simulink library "starslibMathOperations"  (R2024b)
settings: Solver=ode45  StartTime=0.0  StopTime=10.0  RelTol=1e-3  EnableMultiTasking=on
libraries: $bdroot x8
(part 2 of 2)

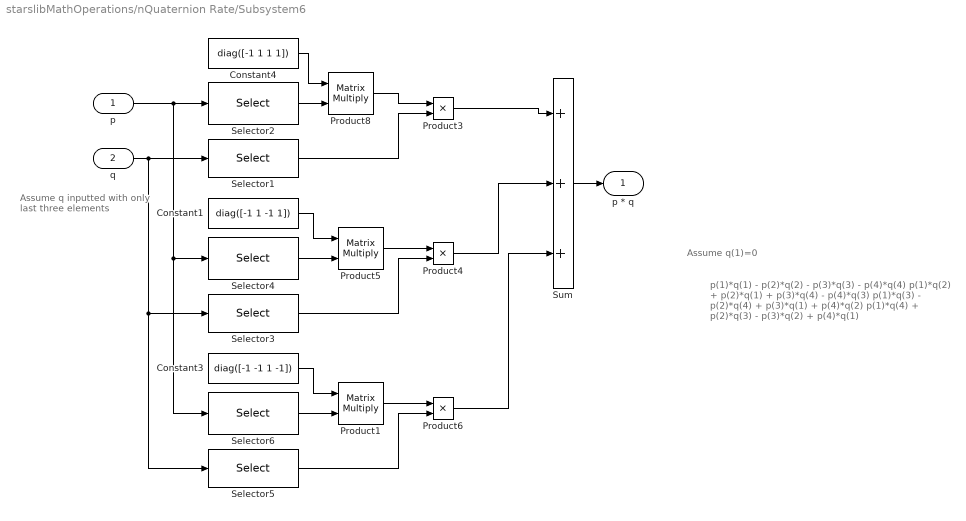
== system starslibMathOperations/nQuaternion Rate/Subsystem6 ==
  note: Assume q
      | inputted with only
      | last three elements
  note: Assume q(1)=0
  note: p(1)*q(1) - p(2)*q(2) - p(3)*q(3) - p(4)*q(4)
      |
      | p(1)*q(2) + p(2)*q(1) + p(3)*q(4) - p(4)*q(3)
      |
      | p(1)*q(3) - p(2)*q(4) + p(3)*q(1) + p(4)*q(2)
      |
      | p(1)*q(4) + p(2)*q(3) - p(3)*q(2) + p(4)*q(1)
  p : Inport  PortDimensions=[4,nQuat]
  q : Inport  Port=2  PortDimensions=[3,nQuat]
  Constant1 : Constant  Value=diag([-1 1 -1 1])  VectorParams1D=off
  Constant3 : Constant  Value=diag([-1 -1 1 -1])  VectorParams1D=off
  Constant4 : Constant  Value=diag([-1 1 1 1])  VectorParams1D=off
  Product1 : Product  Multiplication=Matrix(*)  RndMeth=Zero
  Product3 : Product  RndMeth=Zero
  Product4 : Product  RndMeth=Zero
  Product5 : Product  Multiplication=Matrix(*)  RndMeth=Zero
  Product6 : Product  RndMeth=Zero
  Product8 : Product  Multiplication=Matrix(*)  RndMeth=Zero
  Selector1 : Selector  NumberOfDimensions=2  InputPortWidth=3  IndexOptions=Index vector (dialog),Select all  Indices=[1 1 2 3],1  OutputSizes=1,1
  Selector2 : Selector  NumberOfDimensions=2  InputPortWidth=3  IndexOptions=Index vector (dialog),Select all  Indices=[2 1 1 1],1  OutputSizes=1,1
  Selector3 : Selector  NumberOfDimensions=2  InputPortWidth=3  IndexOptions=Index vector (dialog),Select all  Indices=[2 3 3 2],1  OutputSizes=1,1
  Selector4 : Selector  NumberOfDimensions=2  InputPortWidth=3  IndexOptions=Index vector (dialog),Select all  Indices=[3 3 2 2],1  OutputSizes=1,1
  Selector5 : Selector  NumberOfDimensions=2  InputPortWidth=3  IndexOptions=Index vector (dialog),Select all  Indices=[3 2 1 1],1  OutputSizes=1,1
  Selector6 : Selector  NumberOfDimensions=2  InputPortWidth=3  IndexOptions=Index vector (dialog),Select all  Indices=[4 4 4 3],1  OutputSizes=1,1
  Sum : Sum  Inputs=+++
  p * q : Outport  PortDimensions=[4,nQuat]
  wires:
  Constant4/1 -> Product8/1
  Product8/1 -> Product3/1
  Selector2/1 -> Product8/2
  Sum/1 -> p * q/1
  q/1 -> Selector5/1, Selector3/1, Selector1/1
  p/1 -> Selector6/1, Selector4/1, Selector2/1
  Product6/1 -> Sum/3
  Product4/1 -> Sum/2
  Product3/1 -> Sum/1
  Selector5/1 -> Product6/2
  Product1/1 -> Product6/1
  Selector3/1 -> Product4/2
  Product5/1 -> Product4/1
  Selector1/1 -> Product3/2
  Constant3/1 -> Product1/1
  Selector6/1 -> Product1/2
  Constant1/1 -> Product5/1
  Selector4/1 -> Product5/2

== matlab function starslibMathOperations/funQuaternion Multiplication/Quaternion Multiplication ==
  data: q1 input; q1q2 output; q2 input
function q1q2 = fcn(q1, q2)%#codegen

q1q2 = Qmult(q1,q2);

end
